simulink model "AOO"  (R2020a)
settings: Solver=FixedStepAuto  StartTime=0.0  StopTime=10.0  FixedStep=1e-3  RelTol=1e-3  EnableMultiTasking=on
undefined symbols (not defined in the file): D0, D1, D10, D11, D12, D2, D3, D4, D5, D7, D8, D9, PTA0, PTA1, PTA2, PTB23, PTB9, PTC16, PTC17, PTC3, PTC4, PTD0, PTD2, PTD3
libraries: frdmk64flib x12
settings Model: ExtModeTrigDuration=5  Creator=logan_duui82v  LastModifiedBy=logan_duui82v
settings OptimizationCC: EnhancedBackFolding=on  PassReuseOutputArgsAs=Individual arguments  ZeroExternalMemoryAtStartup=off  ZeroInternalMemoryAtStartup=off  MaxStackSize=64  OptimizeBlockOrder=speed  DifferentSizesBufferReuse=on  OptimizationCustomize=off  EfficientTunableParamExpr=on
settings DebuggingCC: ParameterTunabilityLossMsg=error
settings HardwareCC: ProdBitPerPointer=32  ProdBitPerSizeT=32  ProdBitPerPtrDiffT=32  ProdLargestAtomicInteger=Long  ProdLargestAtomicFloat=Double  ProdWordSize=32  ProdHWDeviceType=ARM Compatible->ARM Cortex
settings SFSimCC: MATLABDynamicMemAlloc=off
settings RTWCC: SystemTargetFile=ert.tlc  HardwareBoard=NXP FRDM-K64F  TemplateMakefile=ert_default_tmf  Toolchain=GNU Tools for ARM Embedded Processors
settings CodeAppCC: ForceParamTrailComments=on  IgnoreCustomStorageClasses=off  OperatorAnnotations=on  SimulinkDataObjDesc=on  SFDataObjDesc=on  InsertBlockDesc=on

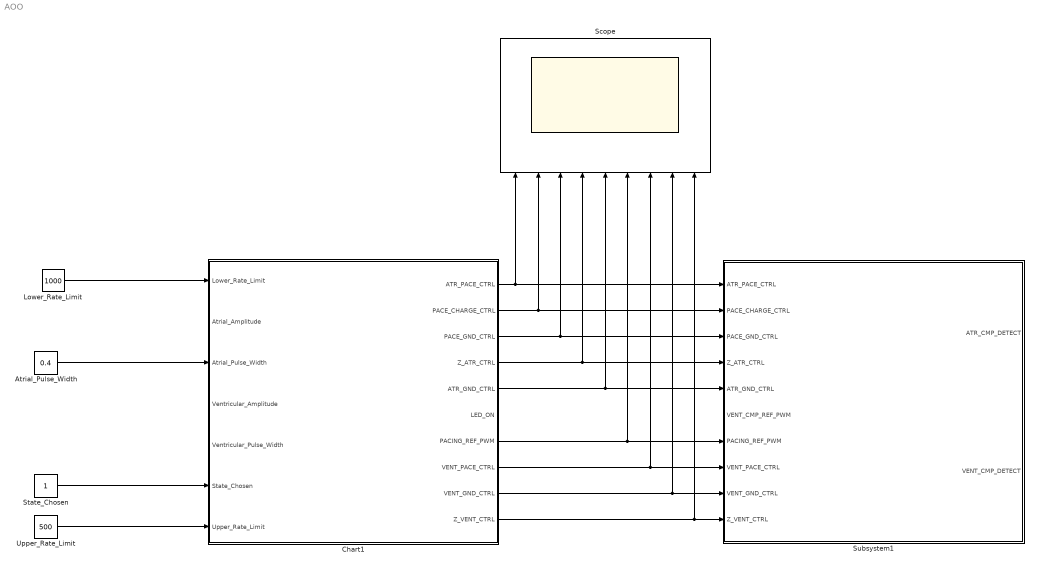
== system AOO ==
  Atrial_Pulse_Width : Constant  Value=0.4  OutDataTypeStr=int32
  Chart1 : Stateflow chart  TreatAsAtomicUnit=on
  Lower_Rate_Limit : Constant  Value=1000  OutDataTypeStr=int32
  Scope : Scope  NumInputPorts=9
  State_Chosen : Constant  OutDataTypeStr=int32
  Subsystem1 : Subsystem
  Upper_Rate_Limit : Constant  Value=500  OutDataTypeStr=int32
  wires:
  State_Chosen/1 -> Chart1/6(State_Chosen)
  Atrial_Pulse_Width/1 -> Chart1/3(Atrial_Pulse_Width)
  Lower_Rate_Limit/1 -> Chart1/1(Lower_Rate_Limit)
  Chart1/1(ATR_PACE_CTRL) -> Subsystem1/1(ATR_PACE_CTRL), Scope/1
  Upper_Rate_Limit/1 -> Chart1/7(Upper_Rate_Limit)
  Chart1/2(PACE_CHARGE_CTRL) -> Subsystem1/2(PACE_CHARGE_CTRL), Scope/2
  Chart1/3(PACE_GND_CTRL) -> Subsystem1/3(PACE_GND_CTRL), Scope/3
  Chart1/4(Z_ATR_CTRL) -> Subsystem1/4(Z_ATR_CTRL), Scope/4
  Chart1/5(ATR_GND_CTRL) -> Subsystem1/5(ATR_GND_CTRL), Scope/5
  Chart1/7(PACING_REF_PWM) -> Subsystem1/7(PACING_REF_PWM), Scope/6
  Chart1/8(VENT_PACE_CTRL) -> Subsystem1/8(VENT_PACE_CTRL), Scope/7
  Chart1/9(VENT_GND_CTRL) -> Subsystem1/9(VENT_GND_CTRL), Scope/8
  Chart1/10(Z_VENT_CTRL) -> Subsystem1/10(Z_VENT_CTRL), Scope/9

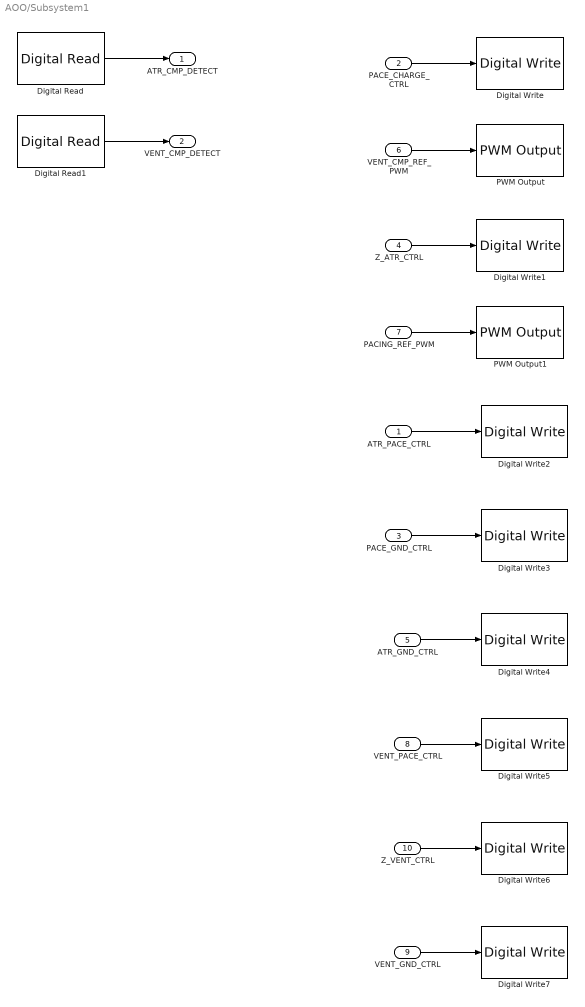
== system AOO/Subsystem1 ==
  ATR_PACE_CTRL : Inport
  PACE_CHARGE_CTRL : Inport  Port=2
  PACE_GND_CTRL : Inport  Port=3
  Z_ATR_CTRL : Inport  Port=4
  ATR_GND_CTRL : Inport  Port=5
  VENT_CMP_REF_PWM : Inport  Port=6
  PACING_REF_PWM : Inport  Port=7
  VENT_PACE_CTRL : Inport  Port=8
  VENT_GND_CTRL : Inport  Port=9
  Z_VENT_CTRL : Inport  Port=10
  Digital Read : frdmk64flib/Digital Read  Whichpin=PTC16 (D0)  SampleTime=-1
  Digital Read1 : frdmk64flib/Digital Read  Whichpin=PTC17 (D1)  SampleTime=-1
  Digital Write : frdmk64flib/Digital Write  Whichpin=PTB9 (D2)
  Digital Write1 : frdmk64flib/Digital Write  Whichpin=PTB23 (D4)
  Digital Write2 : frdmk64flib/Digital Write  Whichpin=PTA0 (D8)
  Digital Write3 : frdmk64flib/Digital Write  Whichpin=PTD0 (D10)
  Digital Write4 : frdmk64flib/Digital Write  Whichpin=PTD2 (D11)
  Digital Write5 : frdmk64flib/Digital Write  Whichpin=PTC4 (D9)
  Digital Write6 : frdmk64flib/Digital Write  Whichpin=PTC3 (D7)
  Digital Write7 : frdmk64flib/Digital Write  Whichpin=PTD3 (D12)
  PWM Output : frdmk64flib/PWM Output  Whichpin=PTA1 (D3)  InitialFrequency=2000  InitialDutyCycle=0
  PWM Output1 : frdmk64flib/PWM Output  Whichpin=PTA2 (D5)  InitialFrequency=2000  InitialDutyCycle=60
  ATR_CMP_DETECT : Outport
  " VENT_CMP_DETECT" : Outport  Port=2
  wires:
  Digital Read/1 -> ATR_CMP_DETECT/1
  Digital Read1/1 -> " VENT_CMP_DETECT"/1
  PACE_CHARGE_CTRL/1 -> Digital Write/1
  VENT_CMP_REF_PWM/1 -> PWM Output/1
  Z_ATR_CTRL/1 -> Digital Write1/1
  PACING_REF_PWM/1 -> PWM Output1/1
  ATR_PACE_CTRL/1 -> Digital Write2/1
  PACE_GND_CTRL/1 -> Digital Write3/1
  ATR_GND_CTRL/1 -> Digital Write4/1
  VENT_PACE_CTRL/1 -> Digital Write5/1
  Z_VENT_CTRL/1 -> Digital Write6/1
  VENT_GND_CTRL/1 -> Digital Write7/1

== stateflow chart AOO/Chart1 ==
  state AOO
    state ChargingDischarging
      entry:
      %Charging
      ATR_PACE_CTRL = false;
      VENT_PACE_CTRL = false;
      PACING_REF_PWM = 50;
      PACE_CHARGE_CTRL = true;
      %Discharging
      %PACE_GND_CTRL = true;
      %VENT_PACE_CTRL = false;
      %Z_ATR_CTRL = false;
      %Z_VENT_CTRL = false;
      %ATR_PACE_CTRL = false
      %ATR_GND_CTRL = true;
      %VENT_GND_CTRL = false;
      %LED_ON = false;
    state APacing
      entry:
      PACE_CHARGE_CTRL = false;
      PACE_GND_CTRL = true;
      ATR_PACE_CTRL = true;
      ATR_GND_CTRL = false;
      Z_ATR_CTRL = false;
      Z_VENT_CTRL = false;
      VENT_GND_CTRL = false;
      VENT_PACE_CTRL = false;
      LED_ON = true;
    state Discharging
      entry:
      PACE_GND_CTRL = true;
      VENT_PACE_CTRL = false;
      Z_ATR_CTRL = false;
      Z_VENT_CTRL = false;
      ATR_PACE_CTRL = false
      ATR_GND_CTRL = true;
      VENT_GND_CTRL = false;
      LED_ON = false;
    (default) -> ChargingDischarging
    ChargingDischarging -> APacing : [after(Lower_Rate_Limit, msec)]
    Discharging -> ChargingDischarging
    APacing -> Discharging : [after(Atrial_Pulse_Width,msec)]
  state initialState
  initialState -> ChargingDischarging : [State_Chosen==1]
  (default) -> initialState
  data: Lower_Rate_Limit input int32; Atrial_Amplitude input; Atrial_Pulse_Width input int32; Ventricular_Amplitude input; Ventricular_Pulse_Width input; State_Chosen input int32; ATR_PACE_CTRL output boolean =false; PACE_CHARGE_CTRL output boolean =false; PACE_GND_CTRL output boolean =false; Z_ATR_CTRL output boolean =false; ATR_GND_CTRL output boolean =false; Upper_Rate_Limit input; LED_ON output boolean; PACING_REF_PWM output double; VENT_PACE_CTRL output boolean; PACING_REF_DUTY local; VENT_GND_CTRL output; Z_VENT_CTRL output
